simulink model "CH5_1"  (Simulink 5.0)
settings: Solver=ode23tb  SolverMode=SingleTasking  StartTime=0.0  StopTime=3/60  RelTol=1e-3
libraries: powerlib2 x8, powerlib_extras x2
Description:
  | 高苑科技大學 電機系
  | 電力電子實驗室
settings Model: Creator=徐瑞隆老師  LastModifiedBy=ELECTRONIC  ExtModeTrigMode=oneshot  ExtModeArmWhenConnect=off  TimeSaveName=t  SaveOutput=off  LimitDataPoints=off  UnconnectedInputMsg=none  UnconnectedOutputMsg=none  BooleanDataType=off  RTWTemplateMakefile=grt_unix.tmf

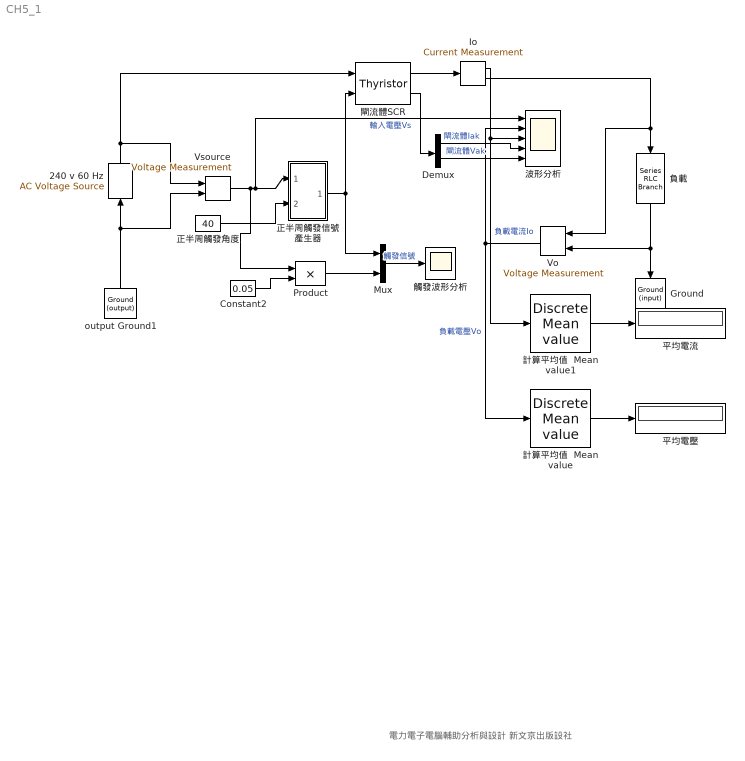
== system CH5_1 ==
  note: 電力電子電腦輔助分析與設計 新文京出版設社
  240 v 60 Hz : powerlib2/Electrical Sources/AC Voltage Source  Tag=PoWeRsYsTeMbLoCk  Orientation=up  A=240*sqrt(2)  P=0  F=60  stime=0  mesure=None  PSBOutputType=1
  Constant2 : Constant  Value=0.05
  Demux : Demux  Outputs=2
  Ground : powerlib2/Connectors/Ground (input)  Tag=PoWeRsYsTeMbLoCk  Orientation=down
  Io : powerlib2/Measurements/Current Measurement  Tag=PoWeRsYsTeMmEaSuReMeNt  PhasorSimulation=off  OutputType=Magnitude  PSBOutputType=01  PSBequivalent=0
  Mux : Mux  Inputs=2
  Product : Product  SaturateOnIntegerOverflow=on  InputSameDT=on
  Vo : powerlib2/Measurements/Voltage Measurement  Tag=PoWeRsYsTeMmEaSuReMeNt  Orientation=left  PhasorSimulation=off  OutputType=Magnitude  PSBOutputType=0  PSBequivalent=0
  Vsource : powerlib2/Measurements/Voltage Measurement  Tag=PoWeRsYsTeMmEaSuReMeNt  PhasorSimulation=off  OutputType=Magnitude  PSBOutputType=0  PSBequivalent=0
  output Ground1 : powerlib2/Connectors/Ground (output)  Tag=PoWeRsYsTeMbLoCk  Orientation=up  PSBOutputType=1
  平均電流 : Display
  平均電壓 : Display
  正半周觸發角度 : Constant  Value=40
  正半周觸發信號 產生器 : Subsystem
  "波形分析 " : Scope  NumInputPorts=5
      settings: TimeRange=0.1  YMin=-50~-100~0~-200~-5  YMax=50~100~40~200~5  DataFormat=Array  MaxDataPoints=2000
  計算平均值  Mean value : powerlib_extras/Discrete Measurements/Discrete  Mean value  AncestorBlock=|  Freq=60  Vinit=0  Ts=50e-6
      | powerlib_extras/Discrete
      | Measurements/Discrete 
      | Mean value
  計算平均值  Mean value1 : powerlib_extras/Discrete Measurements/Discrete  Mean value  AncestorBlock=|  Freq=60  Vinit=0  Ts=50e-6
      | powerlib_extras/Discrete
      | Measurements/Discrete 
      | Mean value
  負載 : powerlib2/Elements/Series RLC Branch  Tag=PoWeRsYsTeMbLoCk  Orientation=down  a=20  b=0e-03  c=inf  mesure=None  PSBOutputType=1
  閘流體SCR : powerlib2/Power Electronics/Thyristor  Tag=PoWeRsYsTeMbLoCk  Ron=1e-3  Lon=0  Vf=0  IC=0  Rs=20000  Cs=1e-9  PSBOutputType=10
  觸發波形分析 : Scope
  wires:
  閘流體SCR/2 -> Demux/1
  閘流體SCR/1 -> Io/1
  Vo/1 -> 計算平均值  Mean value/1, "波形分析 "/2  "負載電壓Vo"
  Io/2 -> Vo/1, 負載/1
  負載/1 -> Ground/1, Vo/2
  Vsource/1 -> 正半周觸發信號 產生器/1(Vs), "波形分析 "/1, Product/1  "輸入電壓Vs"
  output Ground1/1 -> Vsource/2, 240 v 60 Hz/1
  240 v 60 Hz/1 -> Vsource/1, 閘流體SCR/1
  計算平均值  Mean value/1 -> 平均電壓/1
  Mux/1 -> 觸發波形分析/1  "觸發信號"
  Product/1 -> Mux/2
  Constant2/1 -> Product/2
  正半周觸發信號 產生器/1(觸發) -> 閘流體SCR/2, Mux/1
  正半周觸發角度/1 -> 正半周觸發信號 產生器/2(ig1)
  Demux/1 -> "波形分析 "/4  "閘流體Iak"
  Demux/2 -> "波形分析 "/5  "閘流體Vak"
  Io/1 -> "波形分析 "/3, 計算平均值  Mean value1/1  "負載電流Io"
  計算平均值  Mean value1/1 -> 平均電流/1

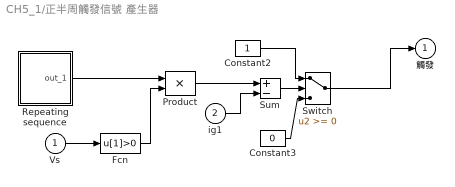
== system CH5_1/正半周觸發信號 產生器 ==
  Vs : Inport
  ig1 : Inport  Port=2
  Constant2 : Constant
  Constant3 : Constant  Value=0
  Fcn : Fcn  Expr=u[1]>0
  Product : Product  SaturateOnIntegerOverflow=on  InputSameDT=on
  Repeating sequence : Subsystem  mask(Repeating table){@1=[0 1/60 ], @2=[0 360 ]}
      mask prompts: @1 "Time values:"; @2 "Output values:"
      mask help:
      | Repeating table.
      | Enter values of time and output for first cycle.
      mask init:
      | period = max(@1); t = @1; y = @2;
      mask Help: Repeats cycle given in table. Time values should be monotonically increasing.
      mask Display: plot([t,t+period,t+2*period],[y,y,y])
  Sum : Sum  Inputs=+-  SaturateOnIntegerOverflow=on  InputSameDT=on
  Switch : Switch  SaturateOnIntegerOverflow=on  InputSameDT=on
  觸發 : Outport  InitialOutput=0
  wires:
  Fcn/1 -> Product/2
  Repeating sequence/1(out_1) -> Product/1
  Constant3/1 -> Switch/3
  Constant2/1 -> Switch/1
  Sum/1 -> Switch/2
  Switch/1 -> 觸發/1
  Product/1 -> Sum/1
  Vs/1 -> Fcn/1
  ig1/1 -> Sum/2

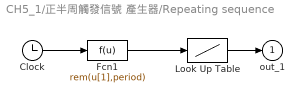
== system CH5_1/正半周觸發信號 產生器/Repeating sequence ==
  Clock : Clock
      settings: Decimation=10
  Fcn1 : Fcn  Expr=rem(u[1],period)
  Look Up Table : Lookup  InputValues=t  OutputValues=y  SaturateOnIntegerOverflow=on
  out_1 : Outport  InitialOutput=0
  wires:
  Fcn1/1 -> Look Up Table/1
  Clock/1 -> Fcn1/1
  Look Up Table/1 -> out_1/1
